simulink model "dvig_3"  (Simulink 9.0)
settings: Solver=ode45  StartTime=0.0  StopTime=4  MaxStep=0.001  MinStep=0.00001  RelTol=1e-3  AbsTol=1e-3  EnableMultiTasking=on
settings Model: SuppressorTable=22 serialization::archive 11 0 6 0 0 0 11 0  Creator=drone  LastModifiedBy=drone
settings DataIOCC: LimitDataPoints=on  SignalLoggingSaveFormat=ModelDataLogs  SaveOutput=off  SaveTime=off  SignalLoggingName=sigsOut
settings OptimizationCC: LifeSpan=auto
settings DebuggingCC: SaveWithParameterizedLinksMsg=none  SignalResolutionControl=TryResolveAllWithWarning  MultiTaskDSMMsg=warning  MultiTaskCondExecSysMsg=none  SFUnexpectedBacktrackingDiag=error  SFNoUnconditionalDefaultTransitionDiag=error  SFExecutionAtInitializationDiag=warning
settings HardwareCC: TargetUnknown=on
settings CodeAppCC: StateflowObjectComments=off
settings GRTTargetCC: CombineOutputUpdateFcns=off  GRTInterface=on

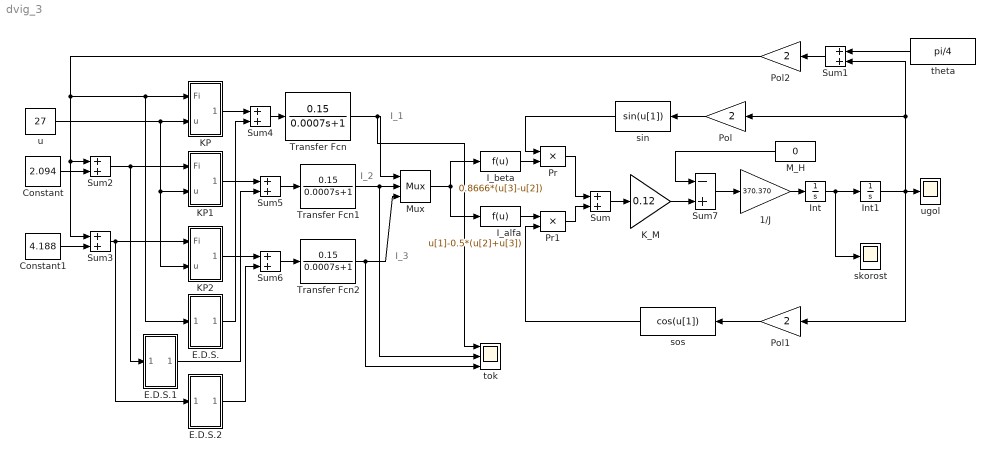
== system dvig_3 ==
  note: I_2
  note: I_1
  note: I_3
  1/J : Gain  Gain=370.370  SaturateOnIntegerOverflow=on  OutDataTypeStr=Inherit: Same as input  ParamDataTypeStr=Inherit: Same as input
  Constant : Constant  Value=2.094
  Constant1 : Constant  Value=4.188
  E.D.S. : Subsystem
  E.D.S.1 : Subsystem
  E.D.S.2 : Subsystem
  I_alfa : Fcn  Expr=u[1]-0.5*(u[2]+u[3])
  I_beta : Fcn  Expr=0.8666*(u[3]-u[2])
  Int : Integrator
  Int1 : Integrator
  KP : Subsystem
  KP1 : Subsystem
  KP2 : Subsystem
  K_M : Gain  Gain=0.12  SaturateOnIntegerOverflow=on  OutDataTypeStr=Inherit: Same as input  ParamDataTypeStr=Inherit: Same as input
  M_H : Constant  Value=0
  Mux : Mux  Inputs=3
  Pol : Gain  Gain=2  SaturateOnIntegerOverflow=on  OutDataTypeStr=Inherit: Same as input  ParamDataTypeStr=Inherit: Same as input
  Pol1 : Gain  Gain=2  SaturateOnIntegerOverflow=on  OutDataTypeStr=Inherit: Same as input  ParamDataTypeStr=Inherit: Same as input
  Pol2 : Gain  Gain=2  SaturateOnIntegerOverflow=on  OutDataTypeStr=Inherit: Same as input  ParamDataTypeStr=Inherit: Same as input
  Pr : Product  SaturateOnIntegerOverflow=on  InputSameDT=on  OutDataTypeStr=Inherit: Same as first input
  Pr1 : Product  SaturateOnIntegerOverflow=on  InputSameDT=on  OutDataTypeStr=Inherit: Same as first input
  Sum{,1..6} (7 alike) : Sum  SaturateOnIntegerOverflow=on  InputSameDT=on  OutDataTypeStr=Inherit: Same as first input
  Sum7 : Sum  Inputs=-+  SaturateOnIntegerOverflow=on  InputSameDT=on  OutDataTypeStr=Inherit: Same as first input
  Transfer Fcn : TransferFcn  Numerator=[0.15]  Denominator=[0.0007 1]
  Transfer Fcn1 : TransferFcn  Numerator=[0.15]  Denominator=[0.0007 1]
  Transfer Fcn2 : TransferFcn  Numerator=[0.15]  Denominator=[0.0007 1]
  sin : Fcn
  skorost : Scope
  sos : Fcn  Expr=cos(u[1])
  theta : Constant  Value=pi/4
  tok : Scope  NumInputPorts=3
  u : Constant  Value=27
  ugol : Scope
  wires:
  I_beta/1 -> Pr/2
  I_alfa/1 -> Pr1/1
  Sum/1 -> K_M/1
  1/J/1 -> Int/1
  Int/1 -> Int1/1, skorost/1
  Pol/1 -> sin/1
  Pol1/1 -> sos/1
  theta/1 -> Sum1/1
  Int1/1 -> Sum1/2, Pol/1, ugol/1, Pol1/1
  Sum1/1 -> Pol2/1
  Constant/1 -> Sum2/2
  u/1 -> KP/2(u), KP1/2(u), KP2/2(u)
  Pol2/1 -> Sum3/1, Sum2/1, KP/1(Fi), E.D.S./1(in_1)
  Constant1/1 -> Sum3/2
  Sum3/1 -> E.D.S.2/1(in_1), KP2/1(Fi)
  Sum4/1 -> Transfer Fcn/1
  KP/1(out_1) -> Sum4/1
  Sum5/1 -> Transfer Fcn1/1
  Sum6/1 -> Transfer Fcn2/1
  KP1/1(out_1) -> Sum5/1
  KP2/1(out_1) -> Sum6/1
  E.D.S./1(out_1) -> Sum4/2
  E.D.S.1/1(out_1) -> Sum5/2
  E.D.S.2/1(out_1) -> Sum6/2
  Pr/1 -> Sum/1
  Pr1/1 -> Sum/2
  Sum7/1 -> 1/J/1
  Sum2/1 -> E.D.S.1/1(in_1), KP1/1(Fi)
  K_M/1 -> Sum7/2
  M_H/1 -> Sum7/1
  sin/1 -> Pr/1
  sos/1 -> Pr1/2
  Transfer Fcn/1 -> tok/1, Mux/1
  Transfer Fcn1/1 -> tok/2, Mux/2
  Transfer Fcn2/1 -> tok/3, Mux/3
  Mux/1 -> I_beta/1, I_alfa/1

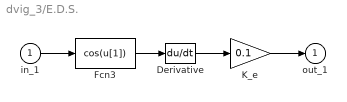
== system dvig_3/E.D.S. ==
  in_1 : Inport
  Derivative : Derivative
  Fcn3 : Fcn  Expr=cos(u[1])
  K_e : Gain  Gain=0.1  SaturateOnIntegerOverflow=on  OutDataTypeStr=Inherit: Same as input  ParamDataTypeStr=Inherit: Same as input
  out_1 : Outport
  wires:
  in_1/1 -> Fcn3/1
  Fcn3/1 -> Derivative/1
  Derivative/1 -> K_e/1
  K_e/1 -> out_1/1

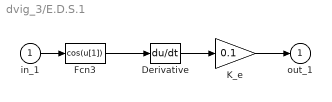
== system dvig_3/E.D.S.1 ==
  in_1 : Inport
  Derivative : Derivative
  Fcn3 : Fcn  Expr=cos(u[1])
  K_e : Gain  Gain=0.1  SaturateOnIntegerOverflow=on  OutDataTypeStr=Inherit: Same as input  ParamDataTypeStr=Inherit: Same as input
  out_1 : Outport
  wires:
  K_e/1 -> out_1/1
  Derivative/1 -> K_e/1
  in_1/1 -> Fcn3/1
  Fcn3/1 -> Derivative/1

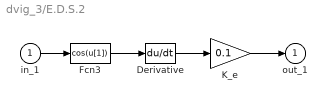
== system dvig_3/E.D.S.2 ==
  in_1 : Inport
  Derivative : Derivative
  Fcn3 : Fcn  Expr=cos(u[1])
  K_e : Gain  Gain=0.1  SaturateOnIntegerOverflow=on  OutDataTypeStr=Inherit: Same as input  ParamDataTypeStr=Inherit: Same as input
  out_1 : Outport
  wires:
  Fcn3/1 -> Derivative/1
  in_1/1 -> Fcn3/1
  Derivative/1 -> K_e/1
  K_e/1 -> out_1/1

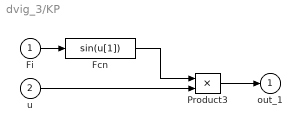
== system dvig_3/KP ==
  Fi : Inport
  u : Inport  Port=2
  Fcn : Fcn
  Product3 : Product  SaturateOnIntegerOverflow=on  InputSameDT=on  OutDataTypeStr=Inherit: Same as first input
  out_1 : Outport
  wires:
  Fi/1 -> Fcn/1
  Product3/1 -> out_1/1
  u/1 -> Product3/2
  Fcn/1 -> Product3/1

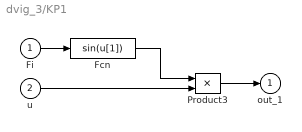
== system dvig_3/KP1 ==
  Fi : Inport
  u : Inport  Port=2
  Fcn : Fcn
  Product3 : Product  SaturateOnIntegerOverflow=on  InputSameDT=on  OutDataTypeStr=Inherit: Same as first input
  out_1 : Outport
  wires:
  Fcn/1 -> Product3/1
  u/1 -> Product3/2
  Product3/1 -> out_1/1
  Fi/1 -> Fcn/1

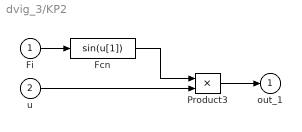
== system dvig_3/KP2 ==
  Fi : Inport
  u : Inport  Port=2
  Fcn : Fcn
  Product3 : Product  SaturateOnIntegerOverflow=on  InputSameDT=on  OutDataTypeStr=Inherit: Same as first input
  out_1 : Outport
  wires:
  Fi/1 -> Fcn/1
  Product3/1 -> out_1/1
  u/1 -> Product3/2
  Fcn/1 -> Product3/1
